simulink model "sys2"  (R2020b)
settings: Solver=VariableStepAuto  StartTime=0.0  StopTime=200  RelTol=1e-3
values from neighbouring files (symbols this model uses):
  A2 = - 1 / (epsilon2 * Td2)    (= -10)    [script.m]
  B2 = [ 1/(epsilon2 * Td2) 0 0]    [script.m]
  C2 = kd2 / epsilon2    (= -2.404)    [script.m]
  d1amp = -0.02    [script.m]
  D2 = [ -k2-kd2/epsilon kr2 -kn2]    [script.m]
  d2amp = 0.04    [script.m]
  hBar = 0    [script.m]
  stateBar = [ hBar; qBar; NBar ]    [script.m]
  uBar = 0    [script.m]
libraries: simulink x2
settings Model: Creator=thoma  LastModifiedBy=thoma

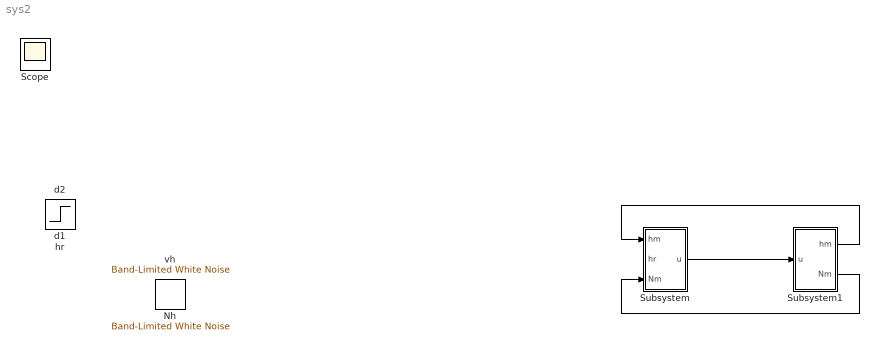
== system sys2 ==
  Subsystem : Subsystem
  Subsystem1 : Subsystem
  Nh : simulink/Sources/Band-Limited White Noise  IOType=siggen  Cov=1e-6  Ts=1e-2  seed=20
  Scope : Scope
  d1 : Step  IOType=siggen  After=d1amp  SampleTime=0
  d2 : Step  IOType=siggen  Time=4  After=d2amp  SampleTime=0
  hr : Step  IOType=siggen  Before=hBar  After=hBar  SampleTime=0
  vh : simulink/Sources/Band-Limited White Noise  IOType=siggen  Cov=1e-6  Ts=1e-2  seed=10
  wires:
  Subsystem/1(u) -> Subsystem1/1(u)
  Subsystem1/1(hm) -> Subsystem/1(hm)
  Subsystem1/2(Nm) -> Subsystem/3(Nm)

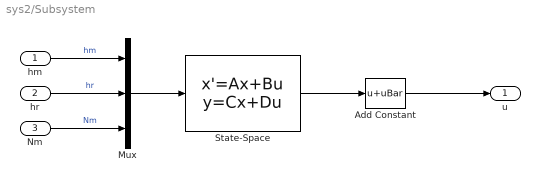
== system sys2/Subsystem ==
  hm : Inport
  hr : Inport  Port=2
  Nm : Inport  Port=3
  Add Constant : Bias  Bias=uBar
  Mux : Mux  Inputs=3
  State-Space : StateSpace  A=A2  B=B2  C=C2  D=D2  InitialCondition=0
  u : Outport
  wires:
  Mux/1 -> State-Space/1
  State-Space/1 -> Add Constant/1
  Add Constant/1 -> u/1
  hm/1 -> Mux/1  "hm"
  hr/1 -> Mux/2  "hr"
  Nm/1 -> Mux/3  "Nm"

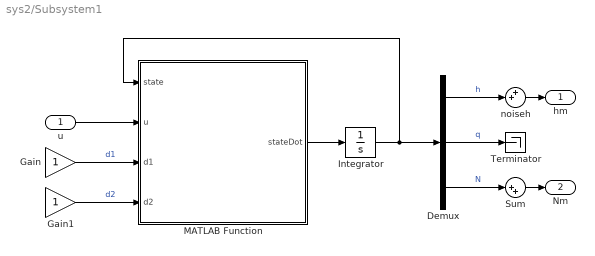
== system sys2/Subsystem1 ==
  u : Inport
  Demux : Demux  Outputs=3
  Gain : Gain
  Gain1 : Gain
  Integrator : Integrator  InitialCondition=stateBar
  MATLAB Function : MATLAB Function  TreatAsAtomicUnit=on
  Sum : Sum  Inputs=|++
  Terminator : Terminator
  noiseh : Sum  Inputs=++|
  hm : Outport
  Nm : Outport  Port=2
  wires:
  Demux/3 -> Sum/1  "N"
  Demux/2 -> Terminator/1  "q"
  noiseh/1 -> hm/1
  Integrator/1 -> MATLAB Function/1(state), Demux/1
  Demux/1 -> noiseh/2  "h"
  MATLAB Function/1(stateDot) -> Integrator/1
  u/1 -> MATLAB Function/2(u)
  Sum/1 -> Nm/1
  Gain/1 -> MATLAB Function/3(d1)  "d1"
  Gain1/1 -> MATLAB Function/4(d2)  "d2"

== matlab function sys2/Subsystem1/MATLAB Function ==
  data: state input; u input; stateDot output; d1 input; d2 input
function stateDot = fcn(state, u, d1, d2)
h = state(1);
q = state(2);
N = state(3);

a = 1.0;
b = 2.5;
c = 0.1;
hBar = 0;
NBar = a/b;

hDot = q;
qDot = b*c*NBar*h - b*(1-c*hBar)*N + d2;
NDot = u + d1;
stateDot = [hDot; qDot; NDot];
